simulink subsystem "PIDantiwindup_sub"  (R2024b)
settings: Solver=VariableStepAuto  StartTime=0.0  StopTime=10.0  RelTol=1e-3
values from neighbouring files (symbols this model uses):
  Kd = Kp*Td    [Plant_EstimTrialUpdateLAB17_04_25.m]
  Ki = Kp/Ti    [Plant_EstimTrialUpdateLAB17_04_25.m]
  Kp = Dk*cos(Dphi)    [Plant_EstimTrialUpdateLAB17_04_25.m]
  Kw = 1/Tw    (= 0.714285714286)    [Plant_EstimTrialUpdateLAB17_04_25.m]
  TL = b * wc    [Plant_EstimTrialUpdateLAB17_04_25.m]
settings Model: Creator=Utente  LastModifiedBy=Riccardo Grosso

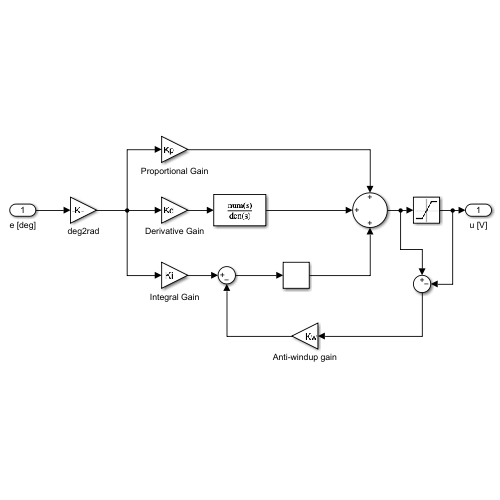
[thumbnail: Simulink's stored preview of the top-level diagram]
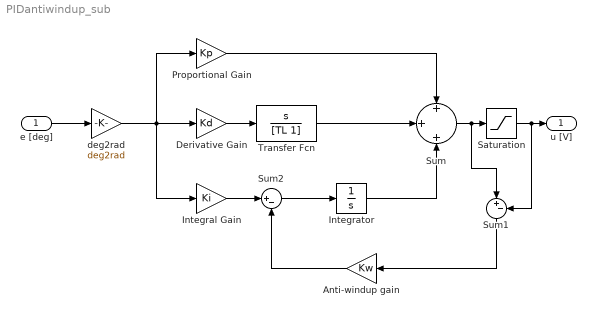
== system PIDantiwindup_sub ==
  e [deg] : Inport
  Anti-windup gain : Gain  Gain=Kw
  Derivative Gain : Gain  Gain=Kd
  Integral Gain : Gain  Gain=Ki
  Integrator : Integrator
  Proportional Gain : Gain  Gain=Kp
  Saturation : Saturate  UpperLimit=+12  LowerLimit=-12
  Sum : Sum  Inputs=+|+|+
  Sum1 : Sum  Inputs=|+-
  Sum2 : Sum  Inputs=|+-
  Transfer Fcn : TransferFcn  Numerator=[1 0]  Denominator=[TL 1]
  deg2rad : Gain  Gain=deg2rad
  u [V] : Outport
  wires:
  Derivative Gain/1 -> Transfer Fcn/1
  e [deg]/1 -> deg2rad/1
  Integral Gain/1 -> Sum2/1
  Anti-windup gain/1 -> Sum2/2
  Proportional Gain/1 -> Sum/1
  Transfer Fcn/1 -> Sum/2
  Sum/1 -> Sum1/1, Saturation/1
  Saturation/1 -> Sum1/2, u [V]/1
  Sum1/1 -> Anti-windup gain/1
  deg2rad/1 -> Integral Gain/1, Derivative Gain/1, Proportional Gain/1
  Sum2/1 -> Integrator/1
  Integrator/1 -> Sum/3
